simulink model "PassiveBalancing_SWC"  (R2024b)
settings: Solver=FixedStepDiscrete  StartTime=0.0  StopTime=200  FixedStep=1e-3  RelTol=1e-3
model workspace (MAT data in the model file):
  Ah = 3
  R = 0.1
  SoC1 = 60
  SoC2 = 70
  SoC3 = 50
  SoC4 = 80
  Vnom = 3.7
settings Model: Creator=MOHAMED  LastModifiedBy=MOHAMED
settings OptimizationCC: DefaultParameterBehavior=Inlined  UseDivisionForNetSlopeComputation=on  GainParamInheritBuiltInType=on  UseFloatMulNetSlope=on  InlineInvariantSignals=on  PassReuseOutputArgsAs=Individual arguments  ZeroExternalMemoryAtStartup=off  ZeroInternalMemoryAtStartup=off  NoFixptDivByZeroProtection=on  EfficientFloat2IntCast=on  LifeSpan=1  OptimizeBlockOrder=speed  DifferentSizesBufferReuse=on  EfficientTunableParamExpr=on
settings DebuggingCC: ParameterTunabilityLossMsg=error
settings HardwareCC: ProdLongLongMode=on
settings SFSimCC: MATLABDynamicMemAlloc=off
settings RTWCC: Description=Embedded Coder  SystemTargetFile=ert.tlc  TemplateMakefile=ert_default_tmf
settings CodeAppCC: ForceParamTrailComments=on  IgnoreCustomStorageClasses=off  OperatorAnnotations=on  SimulinkDataObjDesc=on  SFDataObjDesc=on  CustomSymbolStrGlobalVar=rt$N$M  CustomSymbolStrType=$N$M  CustomSymbolStrFcn=$N$M$F  CustomSymbolStrMacro=$N$M  InsertBlockDesc=on
settings ERTTargetCC: TargetLangStandard=C99 (ISO)  GenerateSampleERTMain=on  IncludeMdlTerminateFcn=off  CombineSignalStateStructs=on  SupportAbsoluteTime=off  SupportComplex=off  SupportNonInlinedSFcns=on  ERTCustomFileTemplate=example_file_process.tlc  ERTFilePackagingFormat=CompactWithDataFile

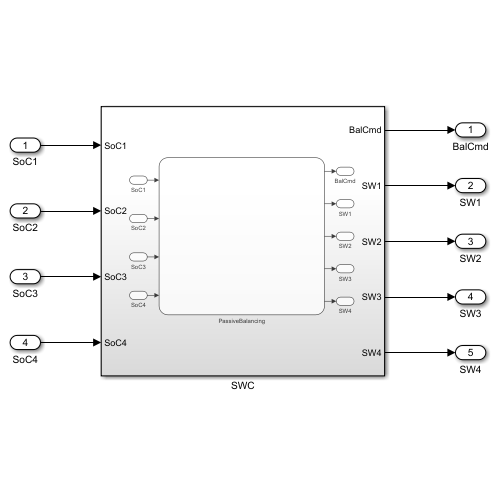
[thumbnail: Simulink's stored preview of the top-level diagram]
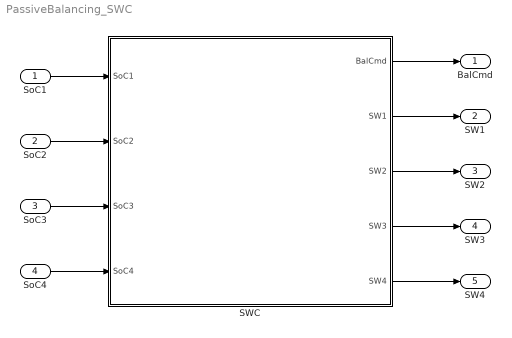
== system PassiveBalancing_SWC ==
  SoC1 : Inport
  SoC2 : Inport  Port=2
  SoC3 : Inport  Port=3
  SoC4 : Inport  Port=4
  SWC : Subsystem
  BalCmd : Outport
  SW1 : Outport  Port=2
  SW2 : Outport  Port=3
  SW3 : Outport  Port=4
  SW4 : Outport  Port=5
  wires:
  SoC1/1 -> SWC/1(SoC1)
  SoC2/1 -> SWC/2(SoC2)
  SWC/4(SW3) -> SW3/1
  SWC/2(SW1) -> SW1/1
  SoC4/1 -> SWC/4(SoC4)
  SWC/3(SW2) -> SW2/1
  SWC/1(BalCmd) -> BalCmd/1
  SWC/5(SW4) -> SW4/1
  SoC3/1 -> SWC/3(SoC3)

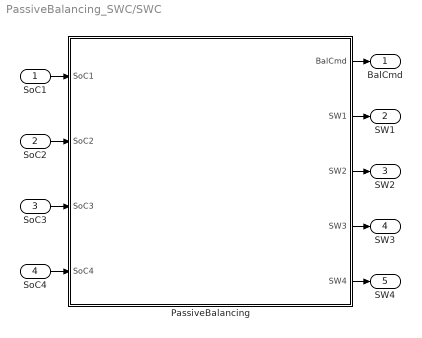
== system PassiveBalancing_SWC/SWC ==
  SoC1 : Inport
  SoC2 : Inport  Port=2
  SoC3 : Inport  Port=3
  SoC4 : Inport  Port=4
  PassiveBalancing : Stateflow chart  TreatAsAtomicUnit=on
  BalCmd : Outport
  SW1 : Outport  Port=2
  SW2 : Outport  Port=3
  SW3 : Outport  Port=4
  SW4 : Outport  Port=5
  wires:
  SoC1/1 -> PassiveBalancing/1(SoC1)
  SoC4/1 -> PassiveBalancing/4(SoC4)
  PassiveBalancing/1(BalCmd) -> BalCmd/1
  PassiveBalancing/2(SW1) -> SW1/1
  SoC3/1 -> PassiveBalancing/3(SoC3)
  PassiveBalancing/3(SW2) -> SW2/1
  PassiveBalancing/4(SW3) -> SW3/1
  SoC2/1 -> PassiveBalancing/2(SoC2)
  PassiveBalancing/5(SW4) -> SW4/1

== stateflow chart PassiveBalancing_SWC/SWC/PassiveBalancing ==
  state BalancingON
    en, du:
    BalCmd = 1;
    Lowest = Min_SoC(SoC1, SoC2, SoC3, SoC4);
    state ControlSW1 [parallel]
      en, du:
      SW1 = ControlSW(SoC1, Lowest);
      settings: executionOrder=1
    state ControlSW2 [parallel]
      en, du:
      SW2 = ControlSW(SoC2, Lowest);
      settings: executionOrder=2
    state ControlSW3 [parallel]
      en, du:
      SW3 = ControlSW(SoC3, Lowest);
      settings: executionOrder=3
    state ControlSW4 [parallel]
      en, du:
      SW4 = ControlSW(SoC4, Lowest);
      settings: executionOrder=4
  state BalancingOFF
    en:
    BalCmd = 0;
  state SW = ControlSW(SoC, Low) [function]
    (default) -> (junction 58) : % Switch Activation
    (junction 58) -> (junction 59) [order 1] : [abs(SoC - Low) > 0.01]
    (junction 58) -> (junction 60) [order 2] : {SW = 0;}
    (junction 59) -> (junction 61) : {SW = 1;}
    (junction 61) -> (junction 60)
    (junction 60) -> (junction 62)
  (default) -> BalancingON
  BalancingON -> BalancingOFF : [BalOFF(SoC1, SoC2, SoC3, SoC4)]
  BalancingOFF -> BalancingON : [~BalOFF(SoC1, SoC2, SoC3, SoC4)]
  data: SoC1 function_input double; SoC2 function_input double; SoC3 function_input double; SoC4 function_input double; out function_output double; SoC1 function_input double; SoC2 function_input double; SoC3 function_input double; SoC4 function_input double; out function_output double; SoC function_input; SW function_output; Low function_input; SoC1 input; SoC2 input; SoC3 input; BalCmd output; SoC4 input; SW1 output; SW2 output; SW3 output; SW4 output; Lowest local
  function out = Min_SoC(SoC1, SoC2, SoC3, SoC4):
    | function out = Min_SoC(SoC1, SoC2, SoC3, SoC4)
    |     out = min(SoC1, min(SoC2, min(SoC3, SoC4)));
    | end
  function out = BalOFF(SoC1, SoC2, SoC3, SoC4):
    | function out = BalOFF(SoC1, SoC2, SoC3, SoC4)
    |     if(abs(SoC1 - SoC2) > 0.001 && abs(SoC1 - SoC3) > 0.001 && abs(SoC1 - SoC4) > 0.001)
    |         out = 1;
    |     else
    |         out = 0;
    |     end
    | end
